simulink model "EnergyEstimationCorrection"  (R2020a)
settings: Solver=FixedStepAuto  StartTime=0  StopTime=time.Time(length(time.Time))  FixedStep=0.10  MaxStep=0.04  RelTol=1e-3
model workspace (MAT data in the model file):
  displayStatus = 1
values from neighbouring files (symbols this model uses):
  routeInfo = 4011    [EnergyEstimationMain.m]
  trip = tripUpdate    [EnergyEstimationMain.m]
undefined symbols (not defined in the file or in its folder): EbatRoute, EdriveRoute, energyDriveActual, energyDriveTrip, energyDriveTripCurrent, eState, massEstimate, sRoute, start, startRoute, stop, stopRoute, timeRoute, vehicleInfo, y, y_Estimate
libraries: simulink x1
(part 2 of 2)

== matlab function EnergyEstimationCorrection/Drivetrain Energy Estimation-Correction ==
  data: timeRoute output; startRoute input; sRoute output; stopRoute input; time input; GPSlat input; GPSlon input; GPShead input; Vx input; s input; Pbat input; Pdrive input; Paux input; Ebat input; Edrive input; Eaux input; EbatRoute output; EdriveRoute output; energyDriveTrip output; energyDriveTripCurrent output; energyDriveActual output; trip parameter; massEstimate output; eState output; y output; y_Estimate output
function [timeRoute, sRoute, EbatRoute, EdriveRoute,energyDriveTrip,energyDriveTripCurrent,energyDriveActual,massEstimate, eState ,y ,y_Estimate] = fcn(startRoute,stopRoute,time,GPSlat,GPSlon,GPShead,Vx,s,Pbat,Pdrive,Paux,Ebat,Edrive,Eaux,trip)

%   Author: Dhruv Jagga
%   Project: Source Code - Cloud Your Bus
%   email: d.jagga@tue.nl
%   Date: 10-12-2019;
%   Revised: 06-08-2020

% Define and Initializing the variables
% Initiated as persistent variables for retaining values of these variables
% to be used in the next time cycle

persistent timeStamp sStamp EbatStamp EdriveStamp P massEstimatePrev

if isempty(timeStamp)
    timeStamp = 0.0;
end

if isempty(sStamp)
    sStamp = 0.0;
end

if isempty(EbatStamp)
    EbatStamp = 0.0;
end

if isempty(EdriveStamp)
    EdriveStamp = 0.0;
end

if isempty(P)
    P = eye(1);
end

if isempty(massEstimatePrev)
    massEstimatePrev = trip.mveh;
end

%%%%%%%%%%%%%%%%%%%%%%%%%%%%%%%%%%%%%%%%%%%%%%%%%%%%%%%%%%%%%%%%%%%%%%%%%%%%%%%%%%%%%%%%%%%%%%%%%%  
% Variable time stamp resetting    

if startRoute == true && stopRoute == false
    timeStamp = time;
    sStamp = s;
    EbatStamp = Ebat;
    EdriveStamp = Edrive;
    massEstimatePrev = trip.mveh;
end

%%%%%%%%%%%%%%%%%%%%%%%%%%%%%%%%%%%%%%%%%%%%%%%%%%%%%%%%%%%%%%%%%%%%%%%%%%%%%%%%%%%%%%%%%%%%%%%%%%  
% Define States
eState1 = 0;
eState2 = 1;

persistent currentState
if isempty(currentState)
    currentState = eState1;
end

eState = currentState;
%%%%%%%%%%%%%%%%%%%%%%%%%%%%%%%%%%%%%%%%%%%%%%%%%%%%%%%%%%%%%%%%%%%%%%%%%%%%%%%%%%%%%%%%%%%%%%%%%%  

% Switch to new state based upon value state register
switch(currentState)
    
    case eState1                        % State when the trip has not yet started
        timeRoute = 0;
        sRoute    = 0;
        EbatRoute = 0;
        EdriveRoute = 0;
        energyDriveTrip= 0;
        energyDriveTripCurrent = 0;
        energyDriveActual= 0;
        massEstimate = trip.mveh;
        y = 0;
        y_Estimate = 0;
        K=0;Q=0;pPrev=0;

%%%%%%%%%%%%%%%%%%%%%%%%%%%%%%%%%%%%%%%%%%%%%%%%%%%%%%%%%%%%%%%%%%%%%%%%%%%%%%%%%%%%%%%%%%%%%%%%%%   
        % State Check
               
        if startRoute == true && stopRoute == false
            currentState = eState2;
        else
            currentState = eState1;
        end

%%%%%%%%%%%%%%%%%%%%%%%%%%%%%%%%%%%%%%%%%%%%%%%%%%%%%%%%%%%%%%%%%%%%%%%%%%%%%%%%%%%%%%%%%%%%%%%%%%  
        
    case eState2                        % State when the trip has started
        timeRoute = time - timeStamp;
        sRoute    = s - sStamp;
        EbatRoute = Ebat - EbatStamp;
        EdriveRoute = Edrive - EdriveStamp;
        
        % Energy estimate powertrain
        EuseEstimate = cumsum(trip.Erate)*massEstimatePrev/3.6e6;                   % Energy estimate in KWh
        EuseFinal    = EuseEstimate(length(EuseEstimate));              % Final energy estimated needed for trip using the previous avg profiles
        EuseCurrent  = interp1(trip.sRoute,EuseEstimate,sRoute);        % Energy usage interpolated with respect to distance travelled
               
        % Total energy consumption estimate for the entire trip
        energyDriveTrip = EuseFinal;                                    % Energy consumtion Estimate given at the start of the trip for entire route
        energyDriveTripCurrent = EuseCurrent;                      
        
        % Actual energy consumption
        energyDriveActual = EdriveRoute;                                % Actual total energy consumed over the trip

%%%%%%%%%%%%%%%%%%%%%%%%%%%%%%%%%%%%%%%%%%%%%%%%%%%%%%%%%%%%%%%%%%%%%%%%%%%%%%%%%%%%%%%%%%%%%%%%%% 
        
        % METHOD 1 - MASS ESTIMATE
        
%         if sRoute > 100
%             energyDiff = (energyActual - EuseCurrent - EuseAuxCurrent);%/EuseCurrent;
%         else
%             energyDiff = 0;
%         end
%         
%         % Vehicle mass estimate for Energy estimate correction;
%         %correctionGain = interp1([0 100 2000 20000],[0 0 0.0005 0.0005],sRoute);
%         correctionGain = interp1([0 100 2000 20000],[0 0 1.2 1.2],sRoute);
%         %massEstimate = mveh*(1 + correctionGain*energyDiff);
%         massEstimate = mveh + correctionGain*energyDiff;
        

%%%%%%%%%%%%%%%%%%%%%%%%%%%%%%%%%%%%%%%%%%%%%%%%%%%%%%%%%%%%%%%%%%%%%%%%%%%%%%%%%%%%%%%%%%%%%%%%%% 

        % METHOD 2 - MASS ESTIMATE (GRADIENT APPROACH)

%         y = (Pbat - Paux);
%         phi = trip.Erate * Vx/3.6e6;
%         
%         phi = phi';
%         
%         yEstimate = phi'*mveh;
%         yEstimate = interp1(trip.s,yEstimate,sRoute);
%         
%         gamma = 1;
%         bias = 1;
%         
%         for i = 1:length(trip.Erate)
%             % Q = sigma;                                         % Unnormalised gradient approach
%             Q = gamma/((abs(phi(i))^2) + bias);                     % Normalised gradient approach
%             
%             K = Q * phi(i);
%         end
%         
%         if sRoute > 100
%             massEstimate = mveh + K * (y - yEstimate);
%         else
%             massEstimate = mveh;
%         end

        % METHOD 2A - MASS ESTIMATE (GRADIENT APPROACH)
        
%         y = EdriveRoute;
%         phi = cumsum(trip.Erate)/3.6e6;
%         
%         phi = phi';
%         
%         yEstimate = phi'*mveh;
%         yEstimate = interp1(trip.sRoute,yEstimate,sRoute);
%         
%         for i = 1:length(trip.Erate)
%             
%             gamma = 1000;
%             bias = 10;
%             Q = sigma;                                         % Unnormalised gradient approach
%             Q = gamma/((abs(phi(i))^2) + bias);                     % Normalised gradient approach
%             
%             K = Q * phi(i);
%         end
%         
%         if sRoute > 100
%             massEstimate = mveh + K * (y - yEstimate);
%         else
%             massEstimate = mveh;
%         end
     
%%%%%%%%%%%%%%%%%%%%%%%%%%%%%%%%%%%%%%%%%%%%%%%%%%%%%%%%%%%%%%%%%%%%%%%%%%%%%%%%%%%%%%%%%%%%%%%%%%    

        % METHOD 3 - MASS ESTIMATE (FORGETTING FACTOR APPROACH)
        
%         y = EdriveRoute;
%         phi = cumsum(trip.Erate)/3.6e6;
%         phi = phi';
%         
%         yEstimate = phi'*mveh;
%         yEstimate = interp1(trip.sRoute,yEstimate,sRoute);
%         
%         for i = 1:length(trip.Erate)
%             lambda = 0.998;
%             pPrev = P;
%             
%             P = (1/lambda)*(pPrev - ((pPrev*(phi(i)*phi(i)')*pPrev)/(lambda + (phi(i)'*pPrev*phi(i)))));
%             Q = pPrev/(lambda + (phi(i)'*pPrev*phi(i)));
%             
%             K = Q * phi(i);
%         end
%         
%         if sRoute > 100
%             massEstimate = mveh + K * (y - yEstimate);
%         else
%             massEstimate = mveh;
%         end

%%%%%%%%%%%%%%%%%%%%%%%%%%%%%%%%%%%%%%%%%%%%%%%%%%%%%%%%%%%%%%%%%%%%%%%%%%%%%%%%%%%%%%%%%%%%%%%%%% 

        % METHOD 4 - MASS ESTIMATE (Kalman Filter Approach)
        
        y = EdriveRoute;
                
        phi = cumsum(trip.Erate)/3.6e6;
        phi = phi';
        
        yEstimate = phi'*massEstimatePrev;
        yEstimate = interp1(trip.sRoute,yEstimate,sRoute);
        
        y_Estimate = yEstimate;
        
        for i = 1:length(trip.Erate)
            R1 = 2.5*1e3;
            R2 = 1;
            pPrev = P;
            
            P = pPrev + R1 - ((pPrev*(phi(i)*phi(i)')*pPrev)/(R2 + (phi(i)'*pPrev*phi(i))));
            Q = pPrev/(R2 + (phi(i)'*pPrev*phi(i)));
            
            K = Q * phi(i);
        end
        
        if sRoute > 100
            massEstimate = massEstimatePrev + K * (y - yEstimate);
        else
            massEstimate = massEstimatePrev;
        end
        
        massEstimatePrev = massEstimate;
        
%%%%%%%%%%%%%%%%%%%%%%%%%%%%%%%%%%%%%%%%%%%%%%%%%%%%%%%%%%%%%%%%%%%%%%%%%%%%%%%%%%%%%%%%%%%%%%%%%%   
        % State Check

        if  startRoute == false && stopRoute == true
            currentState = eState1;
        else
            currentState = eState2;
        end
        
%%%%%%%%%%%%%%%%%%%%%%%%%%%%%%%%%%%%%%%%%%%%%%%%%%%%%%%%%%%%%%%%%%%%%%%%%%%%%%%%%%%%%%%%%%%%%%%%%%

    otherwise
        timeRoute = time;
        sRoute    = s;
        EbatRoute = Ebat;
        EdriveRoute = Edrive;
        energyDriveTrip= 0;
        energyDriveTripCurrent= 0;
        energyDriveActual= 0;
        massEstimate = trip.mveh;
        y = 0;
        y_Estimate = 0;
        K=0;Q=0;pPrev=0;

%%%%%%%%%%%%%%%%%%%%%%%%%%%%%%%%%%%%%%%%%%%%%%%%%%%%%%%%%%%%%%%%%%%%%%%%%%%%%%%%%%%%%%%%%%%%%%%%%%

        
end

== matlab function EnergyEstimationCorrection/Initiate Start Stop ==
  data: time input; GPSlat input; GPSlon input; GPShead input; start parameter; stop parameter; counterStart data_store_memory; startRoute output; stopRoute output; counterStop data_store_memory
function [startRoute, stopRoute] = fcn(time,GPSlat,GPSlon,GPShead,start,stop)

%   Author: Dhruv Jagga
%   Project: Source Code - Cloud Your Bus
%   email: d.jagga@tue.nl
%   Date: 10-12-2019;
%   Revised: 06-08-2020

% Define and Initializing the variables
% Initiated as persistent variables for retaining values of these variables
% to be used in the next time cycle

persistent routeStart routeStop xStart xStop
if isempty(routeStart)
    routeStart = false;                                             % vector which checks if current GPS coordinate is closer to start coordinate
end

if isempty(routeStop)
    routeStop = false;                                              % vector which checks if current GPS coordinate is closer to stop coordinate
end

if isempty(xStart)
    xStart = false;
end

if isempty(xStop)
    xStop = true;
end

global counterStart counterStop

startRoute = false;                                               % checking the number of times the xStart state is active
stopRoute = false;                                                % checking the number of times the xStop state is active

% Storing the values in variable to be used as previous value
routeStart_prev = routeStart;
routeStop_prev = routeStop;

% Compare current GPS coordinate with the specified GPS coordinates of Starting point
if abs(GPSlat - start.lat) < start.latRange && abs(GPSlon - start.lon) < start.lonRange && abs(GPShead - start.head) < start.headRange
    routeStart = true;
    routeStop = false;
    
    if (routeStart_prev == true && routeStart == true) && xStart == false && xStop == true                 % check if 2 consecutive points are closer to start coordinate
        xStart = true;                                                                                     % then raise the flag that route has started
        xStop = false;
        startRoute = xStart;
        
        if xStart == true
            counterStart = counterStart + 1;                                                               % update the route counter
            counterStop = counterStop;
        end
    end
    
% Compare the current GPS coordinate and heading with the Fixed stopping point GPS coordinate
elseif abs(GPSlat - stop.lat) < stop.latRange && abs(GPSlon - stop.lon) < stop.lonRange && abs(GPShead - stop.head) < stop.headRange
    
    routeStart = false;
    routeStop = true;
    
    if (routeStop_prev == true && routeStop == true) && xStart == true && xStop == false                 % check if 2 consecutive points are closer to stop coordinate
        xStart = false;                                                                 % then raise the flag that route has stopped
        xStop = true;
        stopRoute = xStop;
        
        if xStop == true
            counterStop = counterStop + 1;                                              % update the route counter
            counterStart = counterStart;
        end
    end
    
else
% No changes are made if both the conditions are not met
    
    routeStart = false;
    routeStop = false;
end

% Reset counter
if counterStart >= 100 && counterStop >= 100
    counterStart = 0;
    counterStop = 0;
end

end
